simulink model "nonLinearSingleTrack_SchrammHiller_v06"  (R2018b)
settings: Solver=VariableStepAuto  StartTime=0.0  StopTime=5  FixedStep=0.1  RelTol=1e-3
model workspace (MAT data in the model file):
  PCX1 = 1.278793
  PCY1 = 1.38941
  PDX1 = 2.824687
  PDX2 = -0.72384
  PDY1 = -2.509494
  PDY2 = 0.283008
  PKX1 = -60.73047
  PKX2 = 30.18994
  PKX3 = 0.005985
  PKY1 = 73.21113
  T_x = 0.02
  T_y = 0.02
  e_z = 0
  eps = 0.001
  g = 9.81
  h_S = 0.3
  l_h = 0.78
  l_v = 0.77
  m_S = 90
  m_vh = 7.44
  r = 0.26
  theta_vh = 0.4
  theta_zz_vh = 0.22
undefined symbols (not defined in the file): sigbuilder_block
libraries: simulink x1
settings Model: Creator=utente  LastModifiedBy=utente

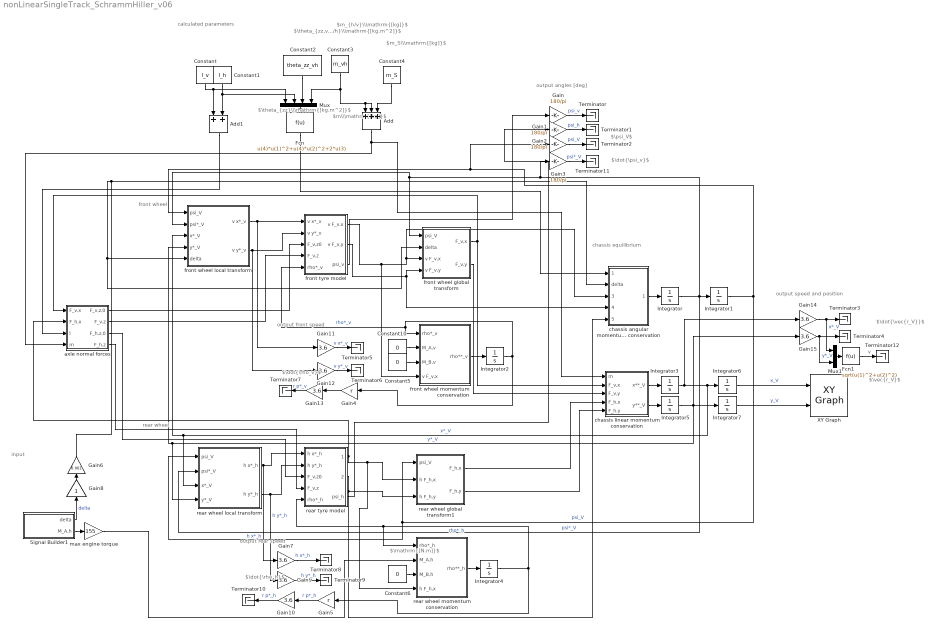
== system nonLinearSingleTrack_SchrammHiller_v06 ==
  note: calculated parameters
  note: output front speed
  note: output angles [deg]
  note: $\mathrm{[N.m]}$
  note: rear wheel
  note: front wheel
  note: chassis equilibrium
  note: output speed and position
  note: $\dot{\rho_h}$
  note: $\dot{\rho_v}$
  note: $\dot{\psi_v}$
  note: $\psi_V$
  note: $\dot{\vec{r_V}}$
  note: $\vec{r_V}$
  note: input
  note: $\theta_{zz,v/h}\\\mathrm{[kg.m^2]}$
  note: $m_{h/v}\\\mathrm{[kg]}$
  note: $m_S\\\mathrm{[kg]}$
  note: $m\\\mathrm{[kg]}$
  note: $\theta_{zz}\\\mathrm{[kg.m^2]}$
  note: output rear speed
  Add : Sum  Inputs=+++
  Add1 : Sum
  Constant : Constant  Value=l_v
  Constant1 : Constant  Value=l_h
  Constant10 : Constant  Value=0
  Constant2 : Constant  Value=theta_zz_vh
  Constant3 : Constant  Value=m_vh
  Constant4 : Constant  Value=m_S
  Constant5 : Constant  Value=0
  Constant6 : Constant  Value=0
  Fcn : Fcn  Expr=u(4)*u(1)^2+u(4)*u(2)^2+2*u(3)
  Fcn1 : Fcn  Expr=sqrt(u(1)^2+u(2)^2)
  Gain{,1..3} (4 alike) : Gain  Gain=180/pi
  Gain{7,9..15} (8 alike) : Gain  Gain=3.6
  Gain4 : Gain  Gain=r
  Gain5 : Gain  Gain=r
  Gain6 : Gain  Gain=0.001
  Gain8 : Gain
  Integrator{,1..7} (8 alike) : Integrator
  Mux : Mux
  Mux1 : Mux  Inputs=2
  Signal Builder1 : Subsystem  Tag=STV Subsys  LoadFcn=sigbuilder_block('load',[150 85.5 433.5 312 ]);  StartFcn=sigbuilder_block('start');  StopFcn=sigbuilder_block('stop');  ClipboardFcn=sigbuilder_block('clipboard');  mask(Sigbuilder block){tuvar=[0:10]}
      mask help: Simulink:masks:SigbuilderBlock_MD
      mask init:
      | if ~strcmp(get_param(bdroot(gcbh),'SimulationStatus'),'stopped') tuvar = sigbuilder_block('maskInit'); end
      settings: CopyFcn=sigbuilder_block('copy');  DeleteFcn=sigbuilder_block('delete');  ModelCloseFcn=sigbuilder_block('modelClose');  PreSaveFcn=sigbuilder_block('preSave');  PauseFcn=sigbuilder_block('pause');  ContinueFcn=sigbuilder_block('continue');  NameChangeFcn=sigbuilder_block('namechange');  OpenFcn=sigbuilder_block('open',[150 85.5 433.5 312 ]);  CloseFcn=sigbuilder_block('close');
      mask Display: plot(0, 0, 100, 100,[2, 2, 32, 32, 2], [68, 8, 8, 68, 68],[32, 2], [38, 38], [32, 19, 2],[53, 60, 44], [32, 17, 17, 2],[16, 16, 31, 31]);txt = getActiveGroup(gcbh);text(2, 100, txt,'verticalAlignment', 'top');
  Terminator{,1..12} (13 alike) : Terminator
  XY Graph : simulink/Sinks/XY Graph  xmin=-20  xmax=40  ymin=-20  ymax=40  st=-1
  axle normal forces : Subsystem
  "chassis angular momentum conservation " : Subsystem
  chassis linear momentum conservation : Subsystem
  front tyre model : Subsystem
  front wheel global transform : Subsystem
  front wheel local transform : Subsystem
  front wheel momentum conservation : Subsystem
  max engine torque : Gain  Gain=155
  rear tyre model : Subsystem
  rear wheel global transform1 : Subsystem
  rear wheel local transform : Subsystem
  rear wheel momentum conservation : Subsystem
  wires:
  Constant3/1 -> Mux/4, Add/2, Add/1
  Constant4/1 -> Add/3
  Mux/1 -> Fcn/1
  Constant2/1 -> Mux/3
  Constant/1 -> Add1/1, Mux/1
  Constant1/1 -> Mux/2, Add1/2
  front tyre model/1(v F_v,x) -> "chassis angular momentum conservation "/3(v F_v,x), front wheel global transform/3(v F_v,x), front wheel momentum conservation/4(v F_v,x)
  Constant10/1 -> front wheel momentum conservation/2(M_A,v)
  front tyre model/2(v F_v,y) -> "chassis angular momentum conservation "/4(v F_v,y), front wheel global transform/4(v F_v,y)
  Integrator/1 -> rear wheel local transform/2(psi*_V), Gain3/1, front wheel local transform/2(psi*_V), front wheel global transform/1(psi_V), Integrator1/1  "psi*_V"
  "chassis angular momentum conservation "/1(psi**_V) -> Integrator/1
  Integrator1/1 -> Gain2/1, front wheel local transform/1(psi_V), rear wheel local transform/1(psi_V), rear wheel global transform1/1(psi_V)  "psi_V"
  Fcn/1 -> "chassis angular momentum conservation "/1(theta_zz)
  front wheel local transform/1(v x*_v) -> Gain11/1, front tyre model/1(v x*_v)
  front wheel local transform/2(v y*_v) -> Gain12/1, front tyre model/2(v y*_v)
  front wheel momentum conservation/1(rho**_v) -> Integrator2/1
  Integrator2/1 -> front tyre model/5(rho*_v), front wheel momentum conservation/1(rho*_v), Gain4/1  "rho*_v"
  Add1/1 -> axle normal forces/3(l)
  axle normal forces/1(F_v,z,0) -> front tyre model/3(F_v,z0)
  axle normal forces/2(F_v,z) -> front tyre model/4(F_v,z)
  front wheel global transform/1(F_v,x) -> axle normal forces/1(F_v,x), chassis linear momentum conservation/2(F_v,x)
  Add/1 -> chassis linear momentum conservation/1(m), axle normal forces/4(m)
  front wheel global transform/2(F_v,y) -> chassis linear momentum conservation/3(F_v,y)
  chassis linear momentum conservation/1(x**_V) -> Integrator3/1
  chassis linear momentum conservation/2(y**_V) -> Integrator5/1
  Integrator3/1 -> Gain14/1, Integrator6/1, rear wheel local transform/3(x*_V), front wheel local transform/3(x*_V)  "x*_V"
  Integrator5/1 -> Gain15/1, Integrator7/1, rear wheel local transform/4(y*_V), front wheel local transform/4(y*_V)  "y*_V"
  rear wheel momentum conservation/1(rho**_h) -> Integrator4/1
  Integrator4/1 -> rear tyre model/5(rho*_h), rear wheel momentum conservation/1(rho*_h), Gain5/1  "rho*_h"
  rear wheel local transform/1(h x*_h) -> Gain7/1, rear tyre model/1(h x*_h)  "h x*_h"
  rear wheel local transform/2(h y*_h) -> Gain9/1, rear tyre model/2(h y*_h)  "h y*_h"
  axle normal forces/3(F_h,z,0) -> rear tyre model/3(F_v,z0)
  axle normal forces/4(F_h,z) -> rear tyre model/4(F_v,z)
  rear tyre model/1(h F_h,x) -> rear wheel momentum conservation/4(h F_h,x), rear wheel global transform1/2(h F_h,x), axle normal forces/2(F_h,x)
  Signal Builder1/1(delta) -> Gain8/1  "delta"
  front tyre model/3(psi_v) -> Gain/1
  rear tyre model/3(psi_h) -> Gain1/1
  Gain/1 -> Terminator/1  "psi_v"
  Gain1/1 -> Terminator1/1  "psi_h"
  Gain2/1 -> Terminator2/1  "psi_V"
  Constant5/1 -> front wheel momentum conservation/3(M_B,v)
  Constant6/1 -> rear wheel momentum conservation/3(M_B,h)
  Integrator7/1 -> XY Graph/2  "y_V"
  Integrator6/1 -> XY Graph/1  "x_V"
  rear wheel global transform1/1(F_h,x) -> chassis linear momentum conservation/4(F_h,x)
  rear wheel global transform1/2(F_h,y) -> chassis linear momentum conservation/5(F_h,y)
  rear tyre model/2(h F_h,y) -> "chassis angular momentum conservation "/5(h F_h,y), rear wheel global transform1/3(h F_h,y)
  Gain4/1 -> Gain13/1
  Gain5/1 -> Gain10/1  "r p*_h"
  Gain3/1 -> Terminator11/1  "psi*_V"
  Gain6/1 -> front wheel global transform/2(delta), front wheel local transform/5(delta), "chassis angular momentum conservation "/2(delta)
  Signal Builder1/2(M_A,h) -> max engine torque/1
  max engine torque/1 -> rear wheel momentum conservation/2(M_A,h)
  Gain8/1 -> Gain6/1
  Gain7/1 -> Terminator8/1  "h x*_h"
  Gain9/1 -> Terminator9/1  "h y*_h"
  Gain10/1 -> Terminator10/1  "r p*_h"
  Gain11/1 -> Terminator5/1  "v x*_v"
  Gain12/1 -> Terminator6/1  "v y*_v"
  Gain13/1 -> Terminator7/1  "r p*_v"
  Gain14/1 -> Mux1/1, Terminator3/1  "x*_V"
  Gain15/1 -> Mux1/2, Terminator4/1  "y*_V"
  Mux1/1 -> Fcn1/1
  Fcn1/1 -> Terminator12/1  "v"

== system nonLinearSingleTrack_SchrammHiller_v06/Signal Builder1 ==
  Demux : Demux  Tag=STV Demux  Outputs=2
  FromWs : FromWorkspace  Tag=STV FromWs  VariableName=tuvar  SampleTime=0
      SigBuilderData=|
      | common.afterFinalStr = 'Extrapolate'
      | common.sampleTime = 0
      | dataSet(1).timeRange = [0 5]
      | dataSet(1).name = 'skidpad'
      | dataSet(2).timeRange = [0 5]
      | dataSet(2).name = 'autocross_2'
      | dataSet(3).timeRange = [0 5]
      | dataSet(3).name = 'accel'
      | dataSet(4).timeRange = [0 5]
      | dataSet(4).name = 'autocross_1'
      | sbobj.Groups(1).Name = 'skidpad'
      | sbobj.Groups(1).Signals(1).Name = 'delta'
      | sbobj.Groups(1).Signals(1).XData = [0 3 3.1 3.2 3.3 3.4 5]
      | sbobj.Groups(1).Signals(1).YData = [0 0 0.028 0.3 0.9 1 1]
      | sbobj.Groups(1).Signals(2).Name = 'M_A,h'
      | sbobj.Groups(1).Signals(2).XData = [0 0.2 0.3 0.4 0.5 2 2.2 2.3 2.4 2.5 5]
      | sbobj.Groups(1).Signals(2).YData = [0 0.2 0.5 0.9 1 1 0.9 0.4 0.1 0 0]
      | sbobj.Groups(1).TimeRange = [0 5]
      | sbobj.Groups(2).Name = 'autocross_2'
      | sbobj.Groups(2).Signals(1).Name = 'delta'
      | sbobj.Groups(2).Signals(1).XData = [0 2.5 2.6 2.7 2.8 3 3.3 3.4 3.5 3.6 3.7 4 4.2 4.3 4.4 5]
      | sbobj.Groups(2).Signals(1).YData = [0 0 0.1 0.5 0.9 1 1 0.9 0 -0.9 -1 -1 -0.9 -0.2 0 0]
      | sbobj.Groups(2).Signals(2).Name = 'M_A,h'
      | sbobj.Groups(2).Signals(2).XData = [0 0.1 0.2 0.3 0.4 0.5 2 2.2 2.3 2.4 2.5 5]
      | sbobj.Groups(2).Signals(2).YData = [0 0.1 0.3 0.7 0.9 1 1 0.9 0.5 0.1 0 0]
      | sbobj.Groups(2).TimeRange = [0 5]
      | sbobj.Groups(3).Name = 'accel'
      | sbobj.Groups(3).Signals(1).Name = 'delta'
      | sbobj.Groups(3).Signals(1).XData = [0 5]
      | sbobj.Groups(3).Signals(1).YData = [0 0]
      | sbobj.Groups(3).Signals(2).Name = 'M_A,h'
      | sbobj.Groups(3).Signals(2).XData = [0 0.1 0.2 0.3 0.4 4.1 4.2 4.3 4.4 4.5 5]
      | sbobj.Groups(3).Signals(2).YData = [0 0.1 0.4 0.9 1 1 0.9 0.5 0.1 0 0]
      | sbobj.Groups(3).TimeRange = [0 5]
      | sbobj.Groups(4).Name = 'autocross_1'
      | sbobj.Groups(4).Signals(1).Name = 'delta'
      | sbobj.Groups(4).Signals(1).XData = [0 3 3.1 3.2 3.3 3.4 3.9 4 4.1 4.2 4.3 5]
      | sbobj.Groups(4).Signals(1).YData = [0 0 0.1 0.3 0.9 1 1 0.9 0.3 0.1 0 0]
      | sbobj.Groups(4).Signals(2).Name = 'M_A,h'
      | sbobj.Groups(4).Signals(2).XData = [0 0.2 0.3 0.4 0.5 2 2.2 2.3 2.4 2.5 5]
      | sbobj.Groups(4).Signals(2).YData = [0 0.2 0.5 0.9 1 1 0.9 0.4 0.1 0 0]
      | sbobj.Groups(4).TimeRange = [0 5]
  delta : Outport  Tag=STV Outport
  M_A,h : Outport  Tag=STV Outport  Port=2
  wires:
  Demux/2 -> M_A,h/1
  FromWs/1 -> Demux/1
  Demux/1 -> delta/1

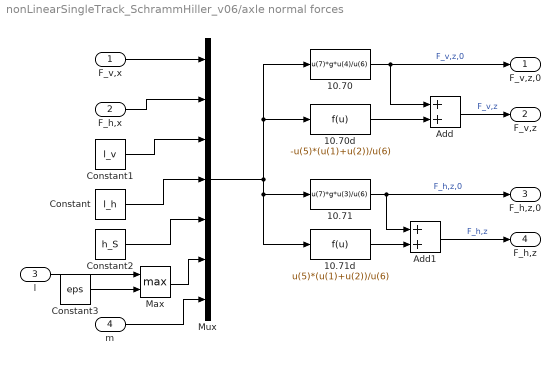
== system nonLinearSingleTrack_SchrammHiller_v06/axle normal forces ==
  F_v,x : Inport
  F_h,x : Inport  Port=2
  l : Inport  Port=3
  m : Inport  Port=4
  10.70 : Fcn  Expr=u(7)*g*u(4)/u(6)
  10.70d : Fcn  Expr=-u(5)*(u(1)+u(2))/u(6)
  10.71 : Fcn  Expr=u(7)*g*u(3)/u(6)
  10.71d : Fcn  Expr=u(5)*(u(1)+u(2))/u(6)
  Add : Sum
  Add1 : Sum
  Constant : Constant  Value=l_h
  Constant1 : Constant  Value=l_v
  Constant2 : Constant  Value=h_S
  Constant3 : Constant  Value=eps
  Max : MinMax  Function=max  Inputs=2
  Mux : Mux  Inputs=7
  F_v,z,0 : Outport
  F_v,z : Outport  Port=2
  F_h,z,0 : Outport  Port=3
  F_h,z : Outport  Port=4
  wires:
  Constant/1 -> Mux/4
  Constant1/1 -> Mux/3
  F_h,x/1 -> Mux/2
  F_v,x/1 -> Mux/1
  Mux/1 -> 10.70/1, 10.70d/1, 10.71d/1, 10.71/1
  Constant2/1 -> Mux/5
  10.70/1 -> Add/1, F_v,z,0/1  "F_v,z,0"
  10.71/1 -> Add1/1, F_h,z,0/1  "F_h,z,0"
  Add/1 -> F_v,z/1  "F_v,z"
  10.70d/1 -> Add/2
  Add1/1 -> F_h,z/1  "F_h,z"
  10.71d/1 -> Add1/2
  m/1 -> Mux/7
  Constant3/1 -> Max/2
  Max/1 -> Mux/6
  l/1 -> Max/1

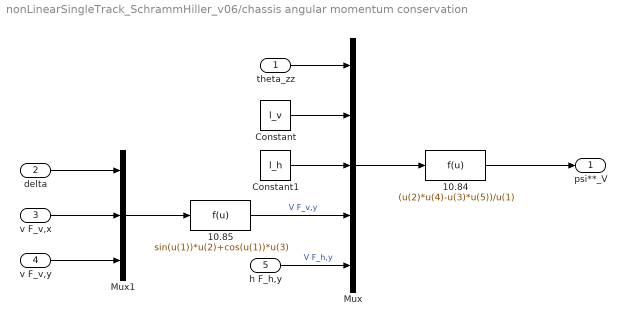
== system nonLinearSingleTrack_SchrammHiller_v06/chassis angular momentum conservation  ==
  theta_zz : Inport
  delta : Inport  Port=2
  v F_v,x : Inport  Port=3
  v F_v,y : Inport  Port=4
  h F_h,y : Inport  Port=5
  10.84 : Fcn  Expr=(u(2)*u(4)-u(3)*u(5))/u(1)
  10.85 : Fcn  Expr=sin(u(1))*u(2)+cos(u(1))*u(3)
  Constant : Constant  Value=l_v
  Constant1 : Constant  Value=l_h
  Mux : Mux  Inputs=5
  Mux1 : Mux  Inputs=3
  psi**_V : Outport
  wires:
  10.84/1 -> psi**_V/1
  Mux/1 -> 10.84/1
  theta_zz/1 -> Mux/1
  Constant/1 -> Mux/2
  Constant1/1 -> Mux/3
  h F_h,y/1 -> Mux/5  "V F_h,y"
  10.85/1 -> Mux/4  "V F_v,y"
  Mux1/1 -> 10.85/1
  delta/1 -> Mux1/1
  v F_v,x/1 -> Mux1/2
  v F_v,y/1 -> Mux1/3

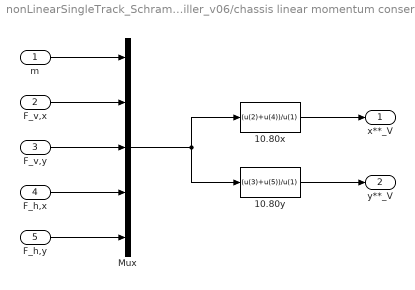
== system nonLinearSingleTrack_SchrammHiller_v06/chassis linear momentum conservation ==
  m : Inport
  F_v,x : Inport  Port=2
  F_v,y : Inport  Port=3
  F_h,x : Inport  Port=4
  F_h,y : Inport  Port=5
  10.80x : Fcn  Expr=(u(2)+u(4))/u(1)
  10.80y : Fcn  Expr=(u(3)+u(5))/u(1)
  Mux : Mux  Inputs=5
  x**_V : Outport
  y**_V : Outport  Port=2
  wires:
  10.80x/1 -> x**_V/1
  10.80y/1 -> y**_V/1
  Mux/1 -> 10.80y/1, 10.80x/1
  m/1 -> Mux/1
  F_v,x/1 -> Mux/2
  F_v,y/1 -> Mux/3
  F_h,x/1 -> Mux/4
  F_h,y/1 -> Mux/5

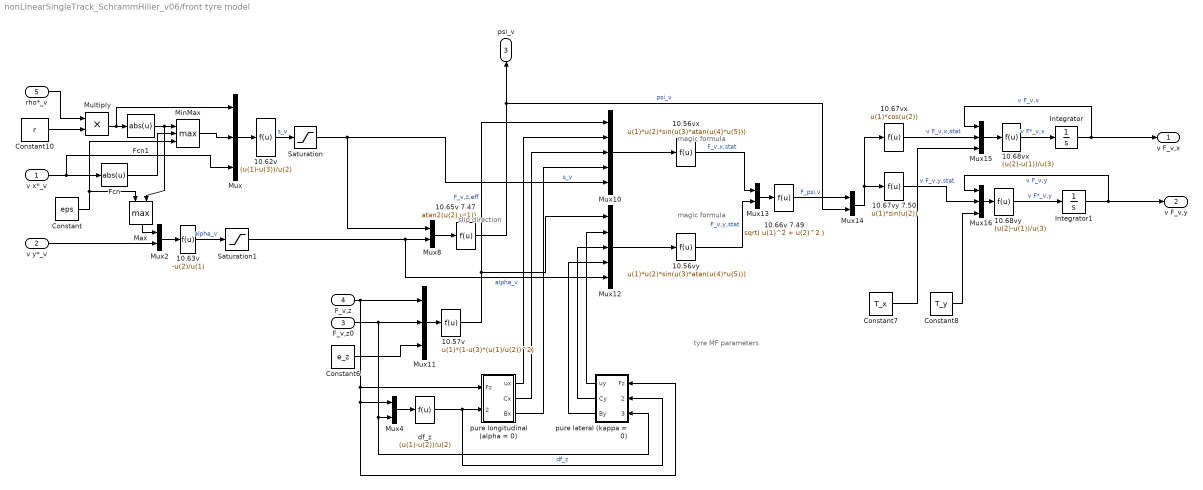
== system nonLinearSingleTrack_SchrammHiller_v06/front tyre model ==
  note: tyre MF parameters
  note: slip direction
  note: magic formula
  note: magic formula
  v x*_v : Inport
  v y*_v : Inport  Port=2
  F_v,z0 : Inport  Port=3
  F_v,z : Inport  Port=4
  rho*_v : Inport  Port=5
  10.56vx : Fcn  Expr=u(1)*u(2)*sin(u(3)*atan(u(4)*u(5)))
  10.56vy : Fcn  Expr=u(1)*u(2)*sin(u(3)*atan(u(4)*u(5)))
  10.57v : Fcn  Expr=u(1)*(1-u(3)*(u(1)/u(2))^2)
  10.62v : Fcn  Expr=(u(1)-u(3))/u(2)
  10.63v : Fcn  Expr=-u(2)/u(1)
  10.65v 7.47 : Fcn  Expr=atan2(u(2),u(1))
  10.66v 7.49 : Fcn  Expr=sqrt( u(1)^2 + u(2)^2 )
  10.67vx : Fcn  Expr=u(1)*cos(u(2))
  10.67vy 7.50 : Fcn  Expr=u(1)*sin(u(2))
  10.68vx : Fcn  Expr=(u(2)-u(1))/u(3)
  10.68vy : Fcn  Expr=(u(2)-u(1))/u(3)
  Constant : Constant  Value=eps
  Constant10 : Constant  Value=r
  Constant6 : Constant  Value=e_z
  Constant7 : Constant  Value=T_x
  Constant8 : Constant  Value=T_y
  Fcn : Fcn  Expr=abs(u)
  Fcn1 : Fcn  Expr=abs(u)
  Integrator : Integrator
  Integrator1 : Integrator
  Max : MinMax  Function=max  Inputs=2
  MinMax : MinMax  Function=max  Inputs=3  ZeroCross=off
  Multiply : Product
  Mux{,11,15..16} (4 alike) : Mux  Inputs=3
  Mux10 : Mux  Inputs=5
  Mux12 : Mux  Inputs=5
  Mux{2,4,8,13..14} (5 alike) : Mux  Inputs=2
  Saturation : Saturate  UpperLimit=0.3  LowerLimit=-0.3  ZeroCross=off
  Saturation1 : Saturate  UpperLimit=15/180*pi  LowerLimit=-15/180*pi  ZeroCross=off
  df_z : Fcn  Expr=(u(1)-u(2))/u(2)
  pure lateral (kappa = 0) : Subsystem
  pure longitudinal (alpha = 0) : Subsystem
  v F_v,x : Outport
  v F_v,y : Outport  Port=2
  psi_v : Outport  Port=3
  wires:
  Mux/1 -> 10.62v/1
  v x*_v/1 -> Mux/3, Fcn/1
  Mux2/1 -> 10.63v/1
  v y*_v/1 -> Mux2/2
  10.65v 7.47/1 -> Mux14/2, psi_v/1  "psi_v"
  Mux8/1 -> 10.65v 7.47/1
  10.63v/1 -> Saturation1/1  "alpha_v"
  Mux10/1 -> 10.56vx/1
  10.56vx/1 -> Mux13/1  "F_v,x,stat"
  Constant6/1 -> Mux11/3
  Mux11/1 -> 10.57v/1
  10.57v/1 -> Mux12/1, Mux10/1  "F_v,z,eff"
  10.56vy/1 -> Mux13/2  "F_v,y,stat"
  Mux12/1 -> 10.56vy/1
  pure lateral (kappa = 0)/1(uy) -> Mux12/2
  pure lateral (kappa = 0)/2(Cy) -> Mux12/3
  pure lateral (kappa = 0)/3(By) -> Mux12/4
  10.62v/1 -> Saturation/1  "s_v"
  Mux13/1 -> 10.66v 7.49/1
  10.66v 7.49/1 -> Mux14/1  "F_psi,v"
  Mux14/1 -> 10.67vx/1, 10.67vy 7.50/1
  10.67vx/1 -> Mux15/2  "v F_v,x,stat"
  10.67vy 7.50/1 -> Mux16/2  "v F_v,y,stat"
  Integrator/1 -> v F_v,x/1, Mux15/1  "v F_v,x"
  Mux15/1 -> 10.68vx/1
  Mux16/1 -> 10.68vy/1
  10.68vx/1 -> Integrator/1  "v F*_v,x"
  10.68vy/1 -> Integrator1/1  "v F*_v,y"
  Integrator1/1 -> v F_v,y/1, Mux16/1  "v F_v,y"
  Constant7/1 -> Mux15/3
  Constant8/1 -> Mux16/3
  pure longitudinal (alpha = 0)/1(ux) -> Mux10/2
  pure longitudinal (alpha = 0)/2(Cx) -> Mux10/3
  pure longitudinal (alpha = 0)/3(Bx) -> Mux10/4
  F_v,z/1 -> pure lateral (kappa = 0)/1(Fz), Mux4/1, pure longitudinal (alpha = 0)/1(Fz), Mux11/1
  Mux4/1 -> df_z/1
  F_v,z0/1 -> Mux4/2, pure lateral (kappa = 0)/3(Fz0), Mux11/2
  df_z/1 -> pure lateral (kappa = 0)/2(df_z), pure longitudinal (alpha = 0)/2(df_z)  "df_z"
  MinMax/1 -> Mux/2
  Fcn/1 -> MinMax/2
  Constant10/1 -> Multiply/2
  rho*_v/1 -> Multiply/1
  Multiply/1 -> Mux/1, Fcn1/1
  Fcn1/1 -> Max/2, MinMax/1
  Constant/1 -> Max/1, MinMax/3
  Max/1 -> Mux2/1
  Saturation1/1 -> Mux12/5, Mux8/2  "alpha_v"
  Saturation/1 -> Mux10/5, Mux8/1  "s_v"

== system nonLinearSingleTrack_SchrammHiller_v06/front wheel global transform ==
  psi_V : Inport
  delta : Inport  Port=2
  v F_v,x : Inport  Port=3
  v F_v,y : Inport  Port=4
  10.82x : Fcn  Expr=cos(u(1))*u(2)-sin(u(1))*u(3)
  10.82y : Fcn  Expr=sin(u(1))*u(2)+cos(u(1))*u(3)
  Add : Sum
  Mux : Mux  Inputs=3
  F_v,x : Outport
  F_v,y : Outport  Port=2
  wires:
  10.82y/1 -> F_v,y/1  "F_v,y"
  10.82x/1 -> F_v,x/1  "F_v,x"
  Mux/1 -> 10.82y/1, 10.82x/1
  v F_v,x/1 -> Mux/2
  v F_v,y/1 -> Mux/3
  Add/1 -> Mux/1
  psi_V/1 -> Add/1
  delta/1 -> Add/2

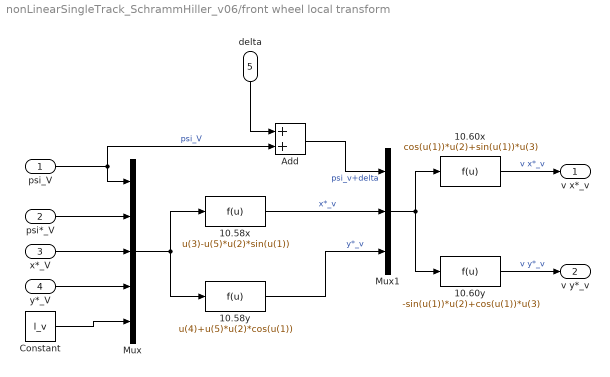
== system nonLinearSingleTrack_SchrammHiller_v06/front wheel local transform ==
  psi_V : Inport
  psi*_V : Inport  Port=2
  x*_V : Inport  Port=3
  y*_V : Inport  Port=4
  delta : Inport  Port=5
  10.58x : Fcn  Expr=u(3)-u(5)*u(2)*sin(u(1))
  10.58y : Fcn  Expr=u(4)+u(5)*u(2)*cos(u(1))
  10.60x : Fcn  Expr=cos(u(1))*u(2)+sin(u(1))*u(3)
  10.60y : Fcn  Expr=-sin(u(1))*u(2)+cos(u(1))*u(3)
  Add : Sum
  Constant : Constant  Value=l_v
  Mux : Mux  Inputs=5
  Mux1 : Mux  Inputs=3
  v x*_v : Outport
  v y*_v : Outport  Port=2
  wires:
  10.58x/1 -> Mux1/2  "x*_v"
  10.58y/1 -> Mux1/3  "y*_v"
  psi_V/1 -> Add/2, Mux/1  "psi_V"
  psi*_V/1 -> Mux/2
  x*_V/1 -> Mux/3
  y*_V/1 -> Mux/4
  Mux/1 -> 10.58x/1, 10.58y/1
  Mux1/1 -> 10.60x/1, 10.60y/1
  Add/1 -> Mux1/1  "psi_v+delta"
  delta/1 -> Add/1
  10.60x/1 -> v x*_v/1  "v x*_v"
  10.60y/1 -> v y*_v/1  "v y*_v"
  Constant/1 -> Mux/5

== system nonLinearSingleTrack_SchrammHiller_v06/front wheel momentum conservation ==
  rho*_v : Inport
  M_A,v : Inport  Port=2
  M_B,v : Inport  Port=3
  v F_v,x : Inport  Port=4
  10.72 (10.86) : Fcn  Expr=(u(2)-u(1)*u(3)-u(6)*u(4))/u(5)
  Constant : Constant  Value=r
  Constant1 : Constant  Value=theta_vh
  Mux : Mux  Inputs=6
  Sign : Signum
  rho**_v : Outport
  wires:
  Mux/1 -> 10.72 (10.86)/1
  10.72 (10.86)/1 -> rho**_v/1
  M_A,v/1 -> Mux/2
  rho*_v/1 -> Sign/1
  Sign/1 -> Mux/1
  M_B,v/1 -> Mux/3
  v F_v,x/1 -> Mux/4
  Constant1/1 -> Mux/5
  Constant/1 -> Mux/6

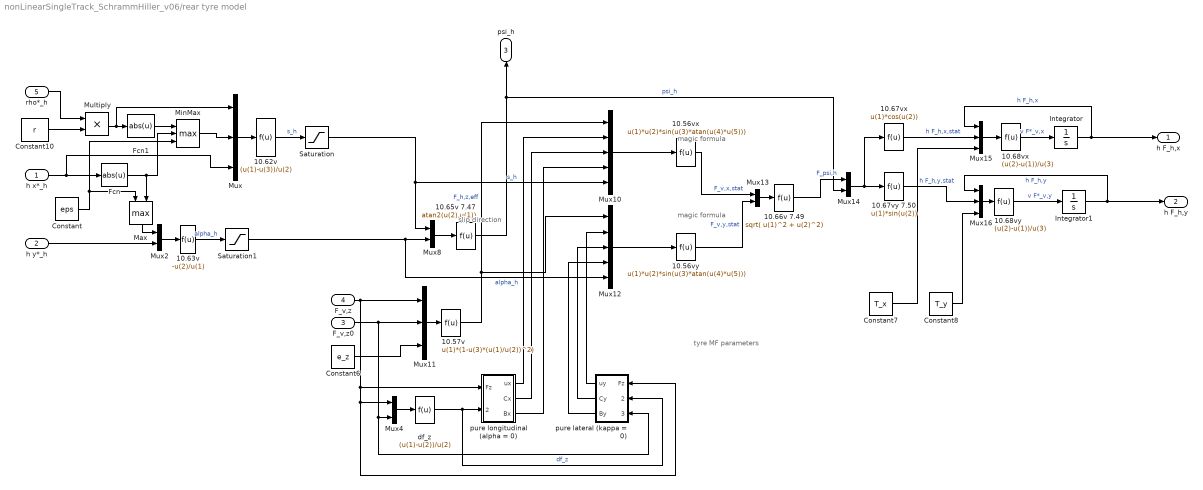
== system nonLinearSingleTrack_SchrammHiller_v06/rear tyre model ==
  note: magic formula
  note: magic formula
  note: slip direction
  note: tyre MF parameters
  h x*_h : Inport
  h y*_h : Inport  Port=2
  F_v,z0 : Inport  Port=3
  F_v,z : Inport  Port=4
  rho*_h : Inport  Port=5
  10.56vx : Fcn  Expr=u(1)*u(2)*sin(u(3)*atan(u(4)*u(5)))
  10.56vy : Fcn  Expr=u(1)*u(2)*sin(u(3)*atan(u(4)*u(5)))
  10.57v : Fcn  Expr=u(1)*(1-u(3)*(u(1)/u(2))^2)
  10.62v : Fcn  Expr=(u(1)-u(3))/u(2)
  10.63v : Fcn  Expr=-u(2)/u(1)
  10.65v 7.47 : Fcn  Expr=atan2(u(2),u(1))
  10.66v 7.49 : Fcn  Expr=sqrt( u(1)^2 + u(2)^2)
  10.67vx : Fcn  Expr=u(1)*cos(u(2))
  10.67vy 7.50 : Fcn  Expr=u(1)*sin(u(2))
  10.68vx : Fcn  Expr=(u(2)-u(1))/u(3)
  10.68vy : Fcn  Expr=(u(2)-u(1))/u(3)
  Constant : Constant  Value=eps
  Constant10 : Constant  Value=r
  Constant6 : Constant  Value=e_z
  Constant7 : Constant  Value=T_x
  Constant8 : Constant  Value=T_y
  Fcn : Fcn  Expr=abs(u)
  Fcn1 : Fcn  Expr=abs(u)
  Integrator : Integrator
  Integrator1 : Integrator
  Max : MinMax  Function=max  Inputs=2
  MinMax : MinMax  Function=max  Inputs=3  ZeroCross=off
  Multiply : Product
  Mux{,11,15..16} (4 alike) : Mux  Inputs=3
  Mux10 : Mux  Inputs=5
  Mux12 : Mux  Inputs=5
  Mux{2,4,8,13..14} (5 alike) : Mux  Inputs=2
  Saturation : Saturate  UpperLimit=0.3  LowerLimit=-0.3  ZeroCross=off
  Saturation1 : Saturate  UpperLimit=15/180*pi  LowerLimit=-15/180*pi  ZeroCross=off
  df_z : Fcn  Expr=(u(1)-u(2))/u(2)
  pure lateral (kappa = 0) : Subsystem
  pure longitudinal (alpha = 0) : Subsystem
  h F_h,x : Outport
  h F_h,y : Outport  Port=2
  psi_h : Outport  Port=3
  wires:
  Max/1 -> Mux2/1
  Constant/1 -> MinMax/3, Max/1
  Fcn1/1 -> MinMax/1
  Multiply/1 -> Fcn1/1, Mux/1
  rho*_h/1 -> Multiply/1
  Constant10/1 -> Multiply/2
  Fcn/1 -> MinMax/2, Max/2
  MinMax/1 -> Mux/2
  df_z/1 -> pure longitudinal (alpha = 0)/2(df_z), pure lateral (kappa = 0)/2(df_z)  "df_z"
  F_v,z0/1 -> Mux11/2, pure lateral (kappa = 0)/3(Fz0), Mux4/2
  Mux4/1 -> df_z/1
  F_v,z/1 -> Mux11/1, pure longitudinal (alpha = 0)/1(Fz), Mux4/1, pure lateral (kappa = 0)/1(Fz)
  pure longitudinal (alpha = 0)/3(Bx) -> Mux10/4
  pure longitudinal (alpha = 0)/2(Cx) -> Mux10/3
  pure longitudinal (alpha = 0)/1(ux) -> Mux10/2
  Constant8/1 -> Mux16/3
  Constant7/1 -> Mux15/3
  Integrator1/1 -> Mux16/1, h F_h,y/1  "h F_h,y"
  10.68vy/1 -> Integrator1/1  "v F*_v,y"
  10.68vx/1 -> Integrator/1  "v F*_v,x"
  Mux16/1 -> 10.68vy/1
  Mux15/1 -> 10.68vx/1
  Integrator/1 -> Mux15/1, h F_h,x/1  "h F_h,x"
  10.67vy 7.50/1 -> Mux16/2  "h F_h,y,stat"
  10.67vx/1 -> Mux15/2  "h F_h,x,stat"
  Mux14/1 -> 10.67vy 7.50/1, 10.67vx/1
  10.66v 7.49/1 -> Mux14/1  "F_psi,h"
  Mux13/1 -> 10.66v 7.49/1
  10.62v/1 -> Saturation/1  "s_h"
  pure lateral (kappa = 0)/3(By) -> Mux12/4
  pure lateral (kappa = 0)/2(Cy) -> Mux12/3
  pure lateral (kappa = 0)/1(uy) -> Mux12/2
  Mux12/1 -> 10.56vy/1
  10.56vy/1 -> Mux13/2  "F_v,y,stat"
  10.57v/1 -> Mux10/1, Mux12/1  "F_h,z,eff"
  Mux11/1 -> 10.57v/1
  Constant6/1 -> Mux11/3
  10.56vx/1 -> Mux13/1  "F_v,x,stat"
  Mux10/1 -> 10.56vx/1
  10.63v/1 -> Saturation1/1  "alpha_h"
  Mux8/1 -> 10.65v 7.47/1
  10.65v 7.47/1 -> Mux14/2, psi_h/1  "psi_h"
  h y*_h/1 -> Mux2/2
  Mux2/1 -> 10.63v/1
  h x*_h/1 -> Fcn/1, Mux/3
  Mux/1 -> 10.62v/1
  Saturation/1 -> Mux10/5, Mux8/1  "s_h"
  Saturation1/1 -> Mux12/5, Mux8/2  "alpha_h"

== system nonLinearSingleTrack_SchrammHiller_v06/rear wheel global transform1 ==
  psi_V : Inport
  h F_h,x : Inport  Port=2
  h F_h,y : Inport  Port=3
  10.83x : Fcn  Expr=cos(u(1))*u(2)-sin(u(1))*u(3)
  10.83y : Fcn  Expr=sin(u(1))*u(2)+cos(u(1))*u(3)
  Mux : Mux  Inputs=3
  F_h,x : Outport
  F_h,y : Outport  Port=2
  wires:
  psi_V/1 -> Mux/1
  h F_h,y/1 -> Mux/3
  h F_h,x/1 -> Mux/2
  Mux/1 -> 10.83x/1, 10.83y/1
  10.83x/1 -> F_h,x/1  "F_h,x"
  10.83y/1 -> F_h,y/1  "F_h,y"

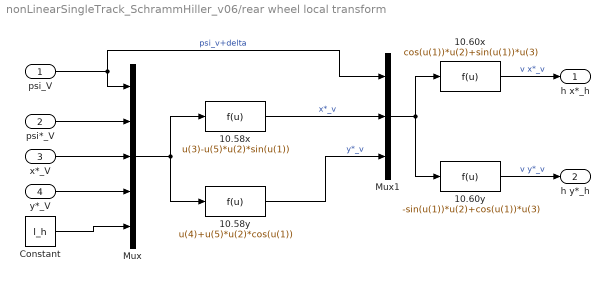
== system nonLinearSingleTrack_SchrammHiller_v06/rear wheel local transform ==
  psi_V : Inport
  psi*_V : Inport  Port=2
  x*_V : Inport  Port=3
  y*_V : Inport  Port=4
  10.58x : Fcn  Expr=u(3)-u(5)*u(2)*sin(u(1))
  10.58y : Fcn  Expr=u(4)+u(5)*u(2)*cos(u(1))
  10.60x : Fcn  Expr=cos(u(1))*u(2)+sin(u(1))*u(3)
  10.60y : Fcn  Expr=-sin(u(1))*u(2)+cos(u(1))*u(3)
  Constant : Constant  Value=l_h
  Mux : Mux  Inputs=5
  Mux1 : Mux  Inputs=3
  h x*_h : Outport
  h y*_h : Outport  Port=2
  wires:
  Constant/1 -> Mux/5
  10.60y/1 -> h y*_h/1  "v y*_v"
  10.60x/1 -> h x*_h/1  "v x*_v"
  psi_V/1 -> Mux1/1, Mux/1  "psi_v+delta"
  Mux1/1 -> 10.60y/1, 10.60x/1
  Mux/1 -> 10.58y/1, 10.58x/1
  y*_V/1 -> Mux/4
  x*_V/1 -> Mux/3
  psi*_V/1 -> Mux/2
  10.58y/1 -> Mux1/3  "y*_v"
  10.58x/1 -> Mux1/2  "x*_v"

== system nonLinearSingleTrack_SchrammHiller_v06/rear wheel momentum conservation ==
  rho*_h : Inport
  M_A,h : Inport  Port=2
  M_B,h : Inport  Port=3
  h F_h,x : Inport  Port=4
  10.72 (10.87) : Fcn  Expr=(u(2)-u(1)*u(3)-u(6)*u(4))/u(5)
  Constant : Constant  Value=r
  Constant1 : Constant  Value=theta_vh
  Mux : Mux  Inputs=6
  Sign : Signum
  rho**_h : Outport
  wires:
  Constant/1 -> Mux/6
  Constant1/1 -> Mux/5
  h F_h,x/1 -> Mux/4
  M_B,h/1 -> Mux/3
  Sign/1 -> Mux/1
  rho*_h/1 -> Sign/1
  M_A,h/1 -> Mux/2
  10.72 (10.87)/1 -> rho**_h/1
  Mux/1 -> 10.72 (10.87)/1

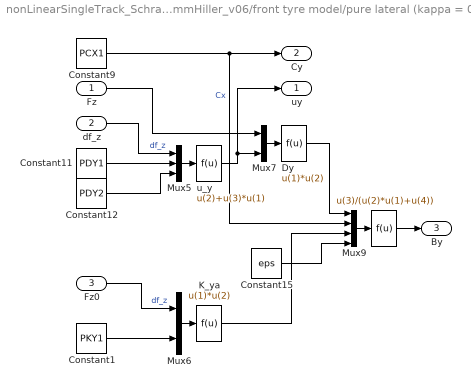
== system nonLinearSingleTrack_SchrammHiller_v06/front tyre model/pure lateral (kappa = 0) ==
  Fz : Inport
  df_z : Inport  Port=2
  Fz0 : Inport  Port=3
  " " : Fcn  Expr=u(3)/(u(2)*u(1)+u(4))
  Constant1 : Constant  Value=PKY1
  Constant11 : Constant  Value=PDY1
  Constant12 : Constant  Value=PDY2
  Constant15 : Constant  Value=eps
  Constant9 : Constant  Value=PCX1
  Dy : Fcn  Expr=u(1)*u(2)
  K_ya : Fcn  Expr=u(1)*u(2)
  Mux5 : Mux  Inputs=3
  Mux6 : Mux  Inputs=2
  Mux7 : Mux  Inputs=2
  Mux9 : Mux
  u_y : Fcn  Expr=u(2)+u(3)*u(1)
  uy : Outport
  Cy : Outport  Port=2
  By : Outport  Port=3
  wires:
  " "/1 -> By/1
  Mux7/1 -> Dy/1
  Constant12/1 -> Mux5/3
  Constant11/1 -> Mux5/2
  Constant1/1 -> Mux6/2
  Mux5/1 -> u_y/1
  Mux9/1 -> " "/1
  Constant9/1 -> Mux9/2, Cy/1  "Cx"
  Constant15/1 -> Mux9/4
  Mux6/1 -> K_ya/1
  Dy/1 -> Mux9/1
  Fz/1 -> Mux7/1
  K_ya/1 -> Mux9/3
  df_z/1 -> Mux5/1  "df_z"
  u_y/1 -> Mux7/2, uy/1
  Fz0/1 -> Mux6/1  "df_z"

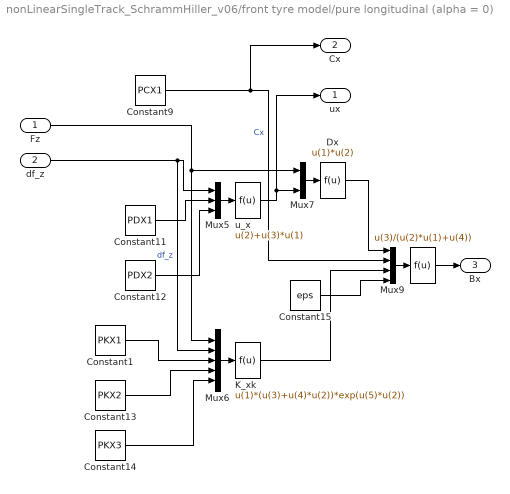
== system nonLinearSingleTrack_SchrammHiller_v06/front tyre model/pure longitudinal (alpha = 0) ==
  Fz : Inport
  df_z : Inport  Port=2
  " " : Fcn  Expr=u(3)/(u(2)*u(1)+u(4))
  Constant1 : Constant  Value=PKX1
  Constant11 : Constant  Value=PDX1
  Constant12 : Constant  Value=PDX2
  Constant13 : Constant  Value=PKX2
  Constant14 : Constant  Value=PKX3
  Constant15 : Constant  Value=eps
  Constant9 : Constant  Value=PCX1
  Dx : Fcn  Expr=u(1)*u(2)
  K_xk : Fcn  Expr=u(1)*(u(3)+u(4)*u(2))*exp(u(5)*u(2))
  Mux5 : Mux  Inputs=3
  Mux6 : Mux  Inputs=5
  Mux7 : Mux  Inputs=2
  Mux9 : Mux
  u_x : Fcn  Expr=u(2)+u(3)*u(1)
  ux : Outport
  Cx : Outport  Port=2
  Bx : Outport  Port=3
  wires:
  u_x/1 -> ux/1, Mux7/2
  df_z/1 -> Mux6/2, Mux5/1  "df_z"
  K_xk/1 -> Mux9/3
  Fz/1 -> Mux7/1, Mux6/1
  Dx/1 -> Mux9/1
  Mux6/1 -> K_xk/1
  Constant15/1 -> Mux9/4
  Constant9/1 -> Cx/1, Mux9/2  "Cx"
  Mux9/1 -> " "/1
  Constant13/1 -> Mux6/4
  Constant14/1 -> Mux6/5
  Mux5/1 -> u_x/1
  Constant1/1 -> Mux6/3
  Constant11/1 -> Mux5/2
  Constant12/1 -> Mux5/3
  Mux7/1 -> Dx/1
  " "/1 -> Bx/1

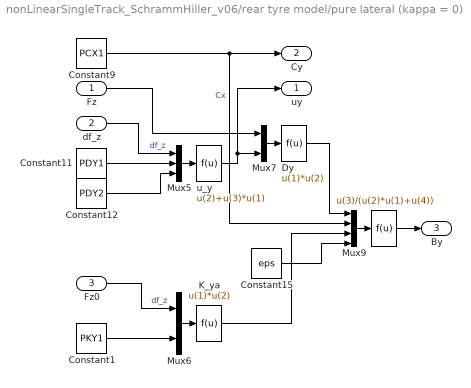
== system nonLinearSingleTrack_SchrammHiller_v06/rear tyre model/pure lateral (kappa = 0) ==
  Fz : Inport
  df_z : Inport  Port=2
  Fz0 : Inport  Port=3
  " " : Fcn  Expr=u(3)/(u(2)*u(1)+u(4))
  Constant1 : Constant  Value=PKY1
  Constant11 : Constant  Value=PDY1
  Constant12 : Constant  Value=PDY2
  Constant15 : Constant  Value=eps
  Constant9 : Constant  Value=PCX1
  Dy : Fcn  Expr=u(1)*u(2)
  K_ya : Fcn  Expr=u(1)*u(2)
  Mux5 : Mux  Inputs=3
  Mux6 : Mux  Inputs=2
  Mux7 : Mux  Inputs=2
  Mux9 : Mux
  u_y : Fcn  Expr=u(2)+u(3)*u(1)
  uy : Outport
  Cy : Outport  Port=2
  By : Outport  Port=3
  wires:
  Fz0/1 -> Mux6/1  "df_z"
  u_y/1 -> uy/1, Mux7/2
  df_z/1 -> Mux5/1  "df_z"
  K_ya/1 -> Mux9/3
  Fz/1 -> Mux7/1
  Dy/1 -> Mux9/1
  Mux6/1 -> K_ya/1
  Constant15/1 -> Mux9/4
  Constant9/1 -> Cy/1, Mux9/2  "Cx"
  Mux9/1 -> " "/1
  Mux5/1 -> u_y/1
  Constant1/1 -> Mux6/2
  Constant11/1 -> Mux5/2
  Constant12/1 -> Mux5/3
  Mux7/1 -> Dy/1
  " "/1 -> By/1

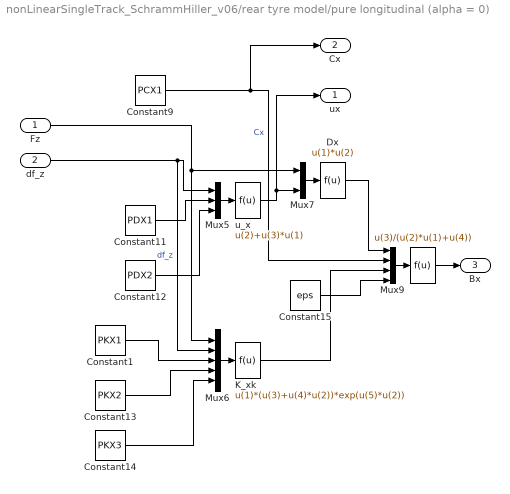
== system nonLinearSingleTrack_SchrammHiller_v06/rear tyre model/pure longitudinal (alpha = 0) ==
  Fz : Inport
  df_z : Inport  Port=2
  " " : Fcn  Expr=u(3)/(u(2)*u(1)+u(4))
  Constant1 : Constant  Value=PKX1
  Constant11 : Constant  Value=PDX1
  Constant12 : Constant  Value=PDX2
  Constant13 : Constant  Value=PKX2
  Constant14 : Constant  Value=PKX3
  Constant15 : Constant  Value=eps
  Constant9 : Constant  Value=PCX1
  Dx : Fcn  Expr=u(1)*u(2)
  K_xk : Fcn  Expr=u(1)*(u(3)+u(4)*u(2))*exp(u(5)*u(2))
  Mux5 : Mux  Inputs=3
  Mux6 : Mux  Inputs=5
  Mux7 : Mux  Inputs=2
  Mux9 : Mux
  u_x : Fcn  Expr=u(2)+u(3)*u(1)
  ux : Outport
  Cx : Outport  Port=2
  Bx : Outport  Port=3
  wires:
  " "/1 -> Bx/1
  Mux7/1 -> Dx/1
  Constant12/1 -> Mux5/3
  Constant11/1 -> Mux5/2
  Constant1/1 -> Mux6/3
  Mux5/1 -> u_x/1
  Constant14/1 -> Mux6/5
  Constant13/1 -> Mux6/4
  Mux9/1 -> " "/1
  Constant9/1 -> Mux9/2, Cx/1  "Cx"
  Constant15/1 -> Mux9/4
  Mux6/1 -> K_xk/1
  Dx/1 -> Mux9/1
  Fz/1 -> Mux6/1, Mux7/1
  K_xk/1 -> Mux9/3
  df_z/1 -> Mux5/1, Mux6/2  "df_z"
  u_x/1 -> Mux7/2, ux/1
